simulink model "verify_DWD_TRY_Radiation_Filter_mdl"  (R2016b)
settings: Solver=VariableStepDiscrete  StartTime=0  StopTime=95*24*3600  MaxStep=60  RelTol=1e-3  EnableMultiTasking=on
InitFcn:
  | load('DE_TRY2010_09_averageYear');
undefined symbols (not defined in the file or in its folder): path_carnot
libraries: carnot x2
settings Model: Creator=drhf  LastModifiedBy=drhf
settings DataIOCC: SaveFormat=Array  SignalLoggingSaveFormat=ModelDataLogs
settings OptimizationCC: ExpressionDepthLimit=2147483647  LifeSpan=inf
settings DebuggingCC: UnderspecifiedInitializationDetection=Classic  MergeDetectMultiDrivingBlocksExec=none  SolverPrmCheckMsg=warning  FcnCallInpInsideContextMsg=warning  StateNameClashWarn=warning  SFUnexpectedBacktrackingDiag=warning  SFNoUnconditionalDefaultTransitionDiag=warning  SFExecutionAtInitializationDiag=none
settings HardwareCC: ProdBitPerPointer=32  ProdBitPerSizeT=32  ProdBitPerPtrDiffT=32  ProdLargestAtomicFloat=None  ProdIntDivRoundTo=Undefined  ProdEndianess=Unspecified  ProdWordSize=32  ProdHWDeviceType=32-bit Generic
settings ModelReferenceCC: PropagateSignalLabelsOutOfModel=off
settings GRTTargetCC: TargetLangStandard=C89/C90 (ANSI)  GeneratePreprocessorConditionals=Disable all  CombineOutputUpdateFcns=off  GRTInterface=on
settings ConfigComp: CovMetricSettings=dw  CovHtmlReporting=on  CovSaveCumulativeToWorkspaceVar=on  CovSaveSingleToWorkspaceVar=on  CovExternalEMLEnable=off

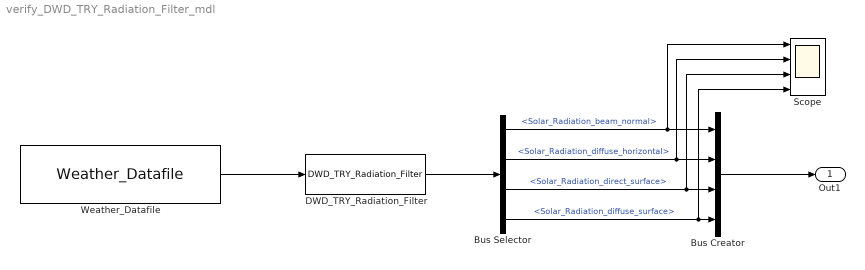
== system verify_DWD_TRY_Radiation_Filter_mdl ==
  Bus Creator : BusCreator  Inputs=4
  Bus Selector : BusSelector  OutputSignals=Solar_Radiation_beam_normal,Solar_Radiation_diffuse_horizontal,Solar_Radiation_direct_surface,Solar_Radiation_diffuse_surface
  DWD_TRY_Radiation_Filter : carnot/Weather/DWD_TRY_Radiation_Filter  f=5
  Scope : Scope  NumInputPorts=4
  Weather_Datafile : carnot/Weather/Weather_Datafile  PathName=path_carnot('data')  FileName='DE_TRY2010_09_averageYear.mat'  UserParam=off  VariableName=DE_TRY2010_09_averageYear  SampleTime=3600
  Out1 : Outport
  wires:
  Bus Selector/2 -> Scope/2, Bus Creator/2  "<Solar_Radiation_diffuse_horizontal>"
  Bus Selector/1 -> Scope/1, Bus Creator/1  "<Solar_Radiation_beam_normal>"
  Bus Creator/1 -> Out1/1
  Weather_Datafile/1 -> DWD_TRY_Radiation_Filter/1
  DWD_TRY_Radiation_Filter/1 -> Bus Selector/1
  Bus Selector/4 -> Scope/4, Bus Creator/4  "<Solar_Radiation_diffuse_surface>"
  Bus Selector/3 -> Scope/3, Bus Creator/3  "<Solar_Radiation_direct_surface>"
